simulink model "stateSpaceToutFait"  (R2015a)
settings: Solver=ode45  StartTime=0.0  StopTime=20  RelTol=1e-3
values from neighbouring files (symbols this model uses):
  A = [0 1; 0 -c/m]    [Untitled2.m]    (also in define_consts.m; loadProperties.m; t.mat = [0  1; 0  -0.025]; test.m)
  B = [0;1/m]    [Untitled2.m]    (also in define_consts.m; loadProperties.m; t.mat = [0 0.1]; test.m = [0 0;1/m 0])
  C = [1 0]    [Untitled2.m]    (also in deadline4.m = tf([4, 1],[0, 2]); define_consts.m; loadProperties.m; t.mat)
  D = 0    [Untitled2.m]    (also in define_consts.m; loadProperties.m; t.mat; test.m = [0 -1])
  K = zeros(1, 2)    [createKL.m]    (also in define_consts.m; test.m = place(A,B,[p1 p2]); test_ref2.m = place(A,B,[p1(i) p2(i)]))
  k_r = K(1)    [createKL.m]    (also in define_consts.m; test_ref2.m = -1/(C*(A-B*K)^-1 *B))
  x0 = [0 0]    [define_consts.m]    (also in loadProperties.m; t.mat = [1 0]; test.m; test_ref2.m = [1 0])
settings Model: Creator=Adrien  LastModifiedBy=Adrien

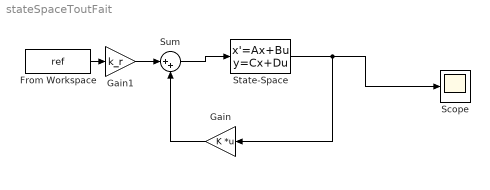
== system stateSpaceToutFait ==
  From Workspace : FromWorkspace  VariableName=ref  SampleTime=step  Interpolate=off  OutputAfterFinalValue=Setting to zero
  Gain : Gain  Gain=K  Multiplication=Matrix(K*u)
  Gain1 : Gain  Gain=k_r
  Scope : Scope
      settings: YMin=0  YMax=100
  State-Space : StateSpace  A=A  B=B  C=C  D=D  X0=x0
  Sum : Sum  Inputs=|++
  wires:
  Gain/1 -> Sum/2
  From Workspace/1 -> Gain1/1
  Gain1/1 -> Sum/1
  State-Space/1 -> Gain/1, Scope/1
  Sum/1 -> State-Space/1
